simulink model "razbijanjePT2"  (R2018b)
settings: Solver=VariableStepAuto  StartTime=0.0  StopTime=10.0  RelTol=1e-3
values from neighbouring files (symbols this model uses):
  w_mm = 19.7845    [LinearizacijaMatrica.m]    (also in Linearizirane_matrice.mat; MPC_designer_X.m = 17; NonTilting.m = 17; RUN_simulation.m = 17)
  zeta_mm = 0.6544    [LinearizacijaMatrica.m]    (also in Linearizirane_matrice.mat; MPC_designer_X.m = 0.85; NonTilting.m = 0.85; RUN_simulation.m = 0.85)
settings Model: Creator=branko  LastModifiedBy=branko

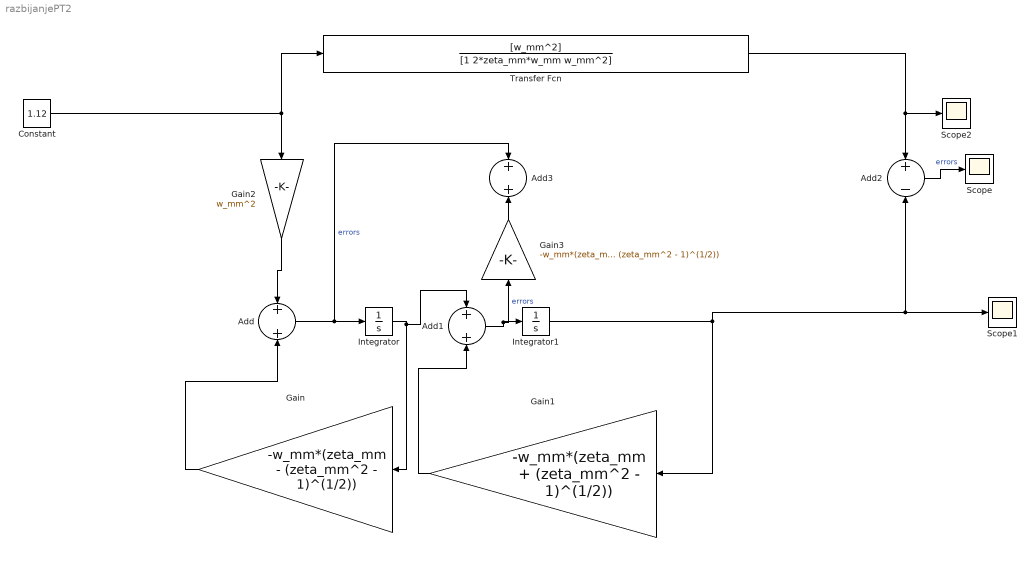
== system razbijanjePT2 ==
  Add : Sum  AccumDataTypeStr=double  OutDataTypeStr=double
  Add1 : Sum  AccumDataTypeStr=double  OutDataTypeStr=double
  Add2 : Sum  Inputs=+-  AccumDataTypeStr=single  OutDataTypeStr=single
  Add3 : Sum  AccumDataTypeStr=double  OutDataTypeStr=double
  Constant : Constant  Value=1.12  OutDataTypeStr=double  SampleTime=-1
  Gain : Gain  Gain=-w_mm*(zeta_mm - (zeta_mm^2 - 1)^(1/2))
  Gain1 : Gain  Gain=-w_mm*(zeta_mm + (zeta_mm^2 - 1)^(1/2))
  Gain2 : Gain  Gain=w_mm^2
  Gain3 : Gain  Gain=-w_mm*(zeta_mm + (zeta_mm^2 - 1)^(1/2))
  Integrator : Integrator
  Integrator1 : Integrator
  Scope : Scope
  Scope1 : Scope
  Scope2 : Scope
  Transfer Fcn : TransferFcn  Numerator=[w_mm^2]  Denominator=[1 2*zeta_mm*w_mm w_mm^2]
  wires:
  Constant/1 -> Gain2/1, Transfer Fcn/1
  Add/1 -> Add3/1, Integrator/1  "errors"
  Integrator/1 -> Add1/1, Gain/1
  Gain/1 -> Add/2
  Gain1/1 -> Add1/2
  Integrator1/1 -> Add2/2, Scope1/1, Gain1/1
  Add1/1 -> Gain3/1, Integrator1/1  "errors"
  Transfer Fcn/1 -> Scope2/1, Add2/1
  Add2/1 -> Scope/1  "errors"
  Gain2/1 -> Add/1
  Gain3/1 -> Add3/2
